simulink model "helicopter_pole_K"  (R2021b)
settings: Solver=ode45  StartTime=0.0  StopTime=T  RelTol=1e-3
InitFcn:
  | hwinit
values from neighbouring files (symbols this model uses):
  A_lin = [0, 1, 0; K1*cos(alpha_ref), -b, -2*K3*omega_ref; 0, 0, -K4 ]    [observer.m]
  B_lin = [0;0; -K4]    [observer.m]
  C = [1, 0, 0; 0, 0, 1]    [MPC_step.m]    (also in contoller_4dim.m; observer.m)
  h = 0.01    [contoller_4dim.m]    (also in observer_check_EKF.m)
  K = place(minssss.A, minssss.B, p_new)    [contoller_4dim.m]
  x_ref = [alpha_ref; alpha_dot_ref; omega_ref;-1]    [contoller_4dim.m]
undefined symbols (not defined in the file or in its folder): adingain, adinoffs, HeliMexHandle
settings Model: Creator=fkzhang  LastModifiedBy=lcaric
settings SolverCC: AlgebraicLoopSolver=TrustRegion
settings DataIOCC: LimitDataPoints=on  SaveFormat=Array  ReturnWorkspaceOutputs=off
settings OptimizationCC: BlockReduction=off  BooleanDataType=off  LifeSpan=inf
settings DebuggingCC: SaveWithParameterizedLinksMsg=none  UnderspecifiedInitializationDetection=Classic  MergeDetectMultiDrivingBlocksExec=none  SignalResolutionControl=TryResolveAllWithWarning  AllowSymbolicDim=off  SFUnexpectedBacktrackingDiag=warning  SFNoUnconditionalDefaultTransitionDiag=warning  SFExecutionAtInitializationDiag=none  SFMachineParentedDataDiag=warning  ArithmeticOperatorsInVariantConditions=warning
settings HardwareCC: ProdBitPerPointer=32  ProdBitPerSizeT=32  ProdBitPerPtrDiffT=32  ProdLargestAtomicFloat=None  ProdIntDivRoundTo=Undefined  ProdEndianess=Unspecified  ProdWordSize=32  ProdHWDeviceType=32-bit Generic  TargetUnknown=on
settings ModelReferenceCC: PropagateSignalLabelsOutOfModel=off
settings SFSimCC: SimUseLocalCustomCode=off  CustomCodeUndefinedFunction=UseInterfaceOnly
settings RTWCC: RTWUseLocalCustomCode=off
settings CodeAppCC: StateflowObjectComments=on
settings GRTTargetCC: TargetLangStandard=C89/C90 (ANSI)
settings ConfigComp: CovMetricSettings=dw  CovSaveCumulativeToWorkspaceVar=on  CovSaveSingleToWorkspaceVar=on  CovExternalEMLEnable=off  CovSFcnEnable=off

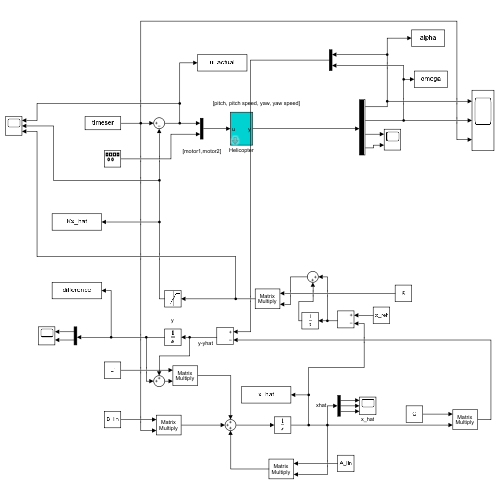
[thumbnail: Simulink's stored preview of the top-level diagram]
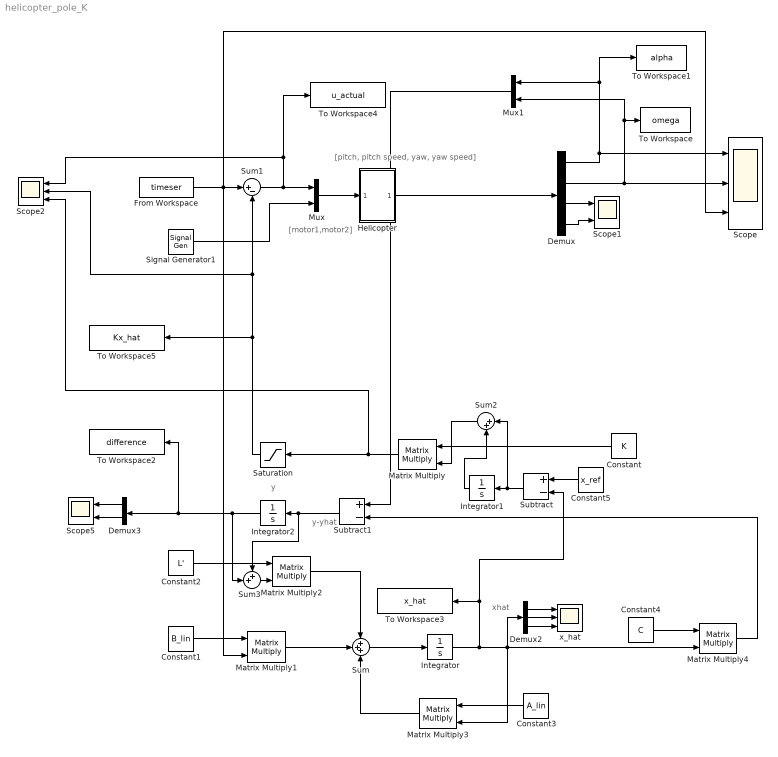
== system helicopter_pole_K ==
  note: y-yhat
  note: y
  note: xhat
  note: [pitch, pitch speed, yaw, yaw speed]
  note: [motor1,motor2]
  Constant : Constant  Value=K  VectorParams1D=off
  Constant1 : Constant  Value=B_lin  VectorParams1D=off
  Constant2 : Constant  Value=L'
  Constant3 : Constant  Value=A_lin
  Constant4 : Constant  Value=C
  Constant5 : Constant  Value=x_ref
  Demux : Demux
  Demux2 : Demux  Outputs=3
  Demux3 : Demux  Outputs=2
  From Workspace : FromWorkspace  VariableName=timeser
  Helicopter : Subsystem  mask{Ts=h}
      mask prompts: Ts "sampletime"
      mask init:
      | sf_heli_init
      mask Display:
      | port_label('input',1,'u');
      | port_label('output',1,'y');
  Integrator : Integrator
  Integrator1 : Integrator
  Integrator2 : Integrator
  Matrix Multiply{,1..4} (5 alike) : Product  Multiplication=Matrix(*)
  Mux : Mux  Inputs=2
  Mux1 : Mux  Inputs=2
  Saturation : Saturate  UpperLimit=1  LowerLimit=-1
  Scope : Scope  NumInputPorts=3
  Scope1 : Scope  NumInputPorts=2
  Scope2 : Scope  NumInputPorts=3
  Scope5 : Scope  NumInputPorts=2
  Signal Generator1 : SignalGenerator  WaveForm=square  Amplitude=0  Frequency=1/20
  Subtract : Sum  Inputs=+-
  Subtract1 : Sum  Inputs=+-
  Sum : Sum  Inputs=+++
  Sum1 : Sum  Inputs=|+-
  Sum2 : Sum  Inputs=|++
  Sum3 : Sum  Inputs=++|
  To Workspace : ToWorkspace  VariableName=omega  SaveFormat=Timeseries  SampleTime=-1
  To Workspace1 : ToWorkspace  VariableName=alpha  SaveFormat=Timeseries  SampleTime=-1
  To Workspace2 : ToWorkspace  VariableName=difference  SaveFormat=Timeseries  SampleTime=-1
  To Workspace3 : ToWorkspace  VariableName=x_hat  SaveFormat=Timeseries  SampleTime=-1
  To Workspace4 : ToWorkspace  VariableName=u_actual  SaveFormat=Timeseries  SampleTime=-1
  To Workspace5 : ToWorkspace  VariableName=Kx_hat  SaveFormat=Timeseries  SampleTime=-1
  x_hat : Scope  NumInputPorts=3
  wires:
  Mux/1 -> Helicopter/1(In1)
  Signal Generator1/1 -> Mux/2
  Demux/2 -> Scope/2, To Workspace/1, Mux1/2
  Demux/3 -> Scope1/1
  Demux/4 -> Scope1/2
  From Workspace/1 -> Sum1/1, Matrix Multiply1/2, Scope/3
  Demux/1 -> To Workspace1/1, Mux1/1, Scope/1
  Mux1/1 -> Subtract1/1
  Helicopter/1(Out1) -> Demux/1
  Matrix Multiply1/1 -> Sum/2
  Matrix Multiply2/1 -> Sum/1
  Sum/1 -> Integrator/1
  Matrix Multiply3/1 -> Sum/3
  Integrator/1 -> To Workspace3/1, Subtract/2, Matrix Multiply3/2, Matrix Multiply4/2, Demux2/1
  Demux2/2 -> x_hat/2
  Demux2/3 -> x_hat/3
  Demux2/1 -> x_hat/1
  Subtract1/1 -> Sum3/1, Integrator2/1
  Matrix Multiply4/1 -> Subtract1/2
  Demux3/2 -> Scope5/2
  Demux3/1 -> Scope5/1
  Constant1/1 -> Matrix Multiply1/1
  Constant2/1 -> Matrix Multiply2/1
  Constant4/1 -> Matrix Multiply4/1
  Constant3/1 -> Matrix Multiply3/1
  Sum1/1 -> To Workspace4/1, Scope2/1, Mux/1
  Constant/1 -> Matrix Multiply/1
  Saturation/1 -> To Workspace5/1, Scope2/2, Sum1/2
  Matrix Multiply/1 -> Saturation/1, Scope2/3
  Constant5/1 -> Subtract/1
  Subtract/1 -> Sum2/1, Integrator1/1
  Integrator1/1 -> Sum2/2
  Sum2/1 -> Matrix Multiply/2
  Integrator2/1 -> Sum3/2, To Workspace2/1, Demux3/1
  Sum3/1 -> Matrix Multiply2/2

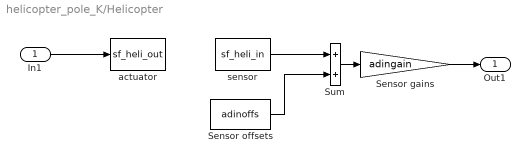
== system helicopter_pole_K/Helicopter ==
  In1 : Inport
  Sensor gains : Gain  Gain=adingain
  Sensor offsets : Constant  Value=adinoffs
  Sum : Sum
  actuator : M-S-Function  FunctionName=sf_heli_out  Parameters=HeliMexHandle,Ts
  sensor : M-S-Function  FunctionName=sf_heli_in  Parameters=HeliMexHandle
  Out1 : Outport  VectorParamsAs1DForOutWhenUnconnected=off
  wires:
  sensor/1 -> Sum/1
  In1/1 -> actuator/1
  Sensor offsets/1 -> Sum/2
  Sum/1 -> Sensor gains/1
  Sensor gains/1 -> Out1/1
